simulink model "ControlNL"  (R2022b)
settings: Solver=ode45  StartTime=0.0  StopTime=1  RelTol=1e-3
values from neighbouring files (symbols this model uses):
  fceq = m*g    (= 20.601)    [Setup.m]
  J = diag([2.85e-6;2.85e-6;1.81e-6])    [Setup.m]
  m = 2.1    [Setup.m]
  MMA = [k1 k1 k1 k1 ... (first row only)    [Setup.m]
  Ts = 0.1    [Setup.m]
  x0 = [p0;v0;q0;omega0]    [Setup.m]
  xlin0 = [p0;v0;alpha0;omega0]    [Setup.m]
libraries: slpidlib x1
settings Model: Creator=stefanotonini  LastModifiedBy=stefanotonini

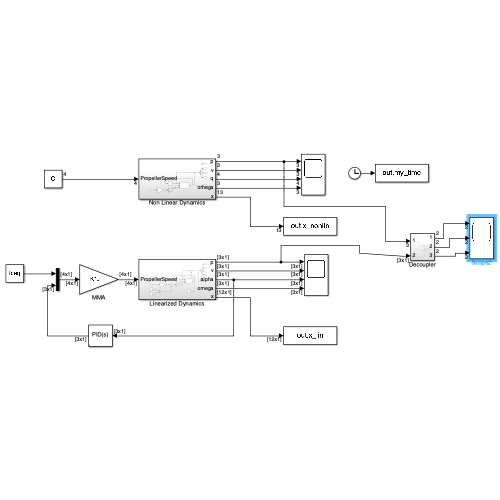
[thumbnail: Simulink's stored preview of the top-level diagram]
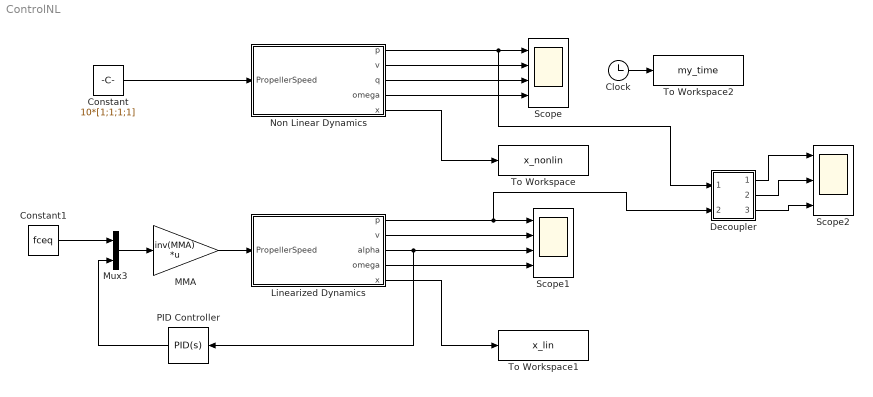
== system ControlNL ==
  Clock : Clock
  Constant : Constant  Value=10*[1;1;1;1]  SampleTime=Ts
  Constant1 : Constant  Value=fceq
  Decoupler : Subsystem
  Linearized Dynamics : Subsystem
  MMA : Gain  Gain=inv(MMA)  Multiplication=Matrix(K*u)
  Mux3 : Mux  Inputs=[1;3]
  Non Linear Dynamics : Subsystem
  PID Controller : slpidlib/PID Controller  Controller=PID  Form=Parallel  TimeDomain=Continuous-time  UseExternalTs=off  SampleTime=-1  IntegratorMethod=Forward Euler  FilterMethod=Forward Euler  ControllerParametersSource=internal  P=1  I=1  UseKiTs=off  D=0  N=100  UseFilter=on  TunerSelectOption=Transfer Function Based (PID Tuner App)  InitialConditionSource=internal  InitialConditionForIntegrator=0  InitialConditionForFilter=0  DifferentiatorICPrevScaledInput=0  ExternalReset=none  TrackingMode=off  Kt=1  LimitOutput=off  SatLimitsSource=internal  UpperSaturationLimit=inf  LowerSaturationLimit=-inf  LinearizeAsGain=on  AntiWindupMode=none  Kb=1  LimitIntegrator=off  UpperIntegratorSaturationLimit=inf  LowerIntegratorSaturationLimit=-inf  POutMin=[]  POutMax=[]  IOutMin=[]  IOutMax=[]  DOutMin=[]  DOutMax=[]  NOutMin=[]  NOutMax=[]  SumOutMin=[]  SumOutMax=[]  SaturationOutMin=[]  SaturationOutMax=[]  PParamMin=[]  PParamMax=[]  IParamMin=[]  IParamMax=[]  DParamMin=[]  DParamMax=[]  NParamMin=[]  NParamMax=[]  KbParamMin=[]  KbParamMax=[]  KtParamMin=[]  KtParamMax=[]  KbOutMin=[]  KbOutMax=[]  KtOutMin=[]  KtOutMax=[]  IntegratorOutMin=[]  IntegratorOutMax=[]  FilterOutMin=[]  FilterOutMax=[]  SumI1OutMin=[]  SumI1OutMax=[]  SumI2OutMin=[]  SumI2OutMax=[]  SumI3OutMin=[]  SumI3OutMax=[]  SumI4OutMin=[]  SumI4OutMax=[]  SumDOutMin=[]  SumDOutMax=[]  DifferentiatorOutMin=[]  DifferentiatorOutMax=[]  FilterDiffOutCoefMin=[]  FilterDiffOutCoefMax=[]  ReciprocalOutMin=[]  ReciprocalOutMax=[]  SumDenOutMin=[]  SumDenOutMax=[]  SumNumOutMin=[]  SumNumOutMax=[]  DivideOutMin=[]  DivideOutMax=[]  UdiffTsProdOutMin=[]  UdiffTsProdOutMax=[]  NTsProdOutMin=[]  NTsProdOutMax=[]  UintegralTsProdOutMin=[]  UintegralTsProdOutMax=[]  UngainTsProdOutMin=[]  UngainTsProdOutMax=[]  ClampingZeroOutDataTypeStr=Inherit: Inherit via back propagation  ClampingZeroOutMin=[]  ClampingZeroOutMax=[]  FilterDenConstantOutDataTypeStr=Inherit: Inherit via back propagation  FilterDenConstantOutMin=[]  FilterDenConstantOutMax=[]  PCopyOutDataTypeStr=Inherit: Inherit via back propagation  PCopyOutMin=[]  PCopyOutMax=[]  NCopyOutDataTypeStr=Inherit: Inherit via back propagation  NCopyOutMin=[]  NCopyOutMax=[]  IntegratorContinuousStateAttributes=''  IntegratorStateMustResolveToSignalObject=off  IntegratorRTWStateStorageClass=Auto  FilterContinuousStateAttributes=''  FilterStateMustResolveToSignalObject=off  FilterRTWStateStorageClass=Auto  ParallelPVariant=InternalParameters  IdealPVariant=Disabled  IVariant=InternalParameters  DVariant=InternalParameters  IntegratorVariant=Continuous  SatVariant=Disabled  AWVariant=Passthrough  PCopyVariant=Disabled  TRVariant=Disabled  FdbkBlocksVariant=Forward  IdealPFdbkVariant=Disabled  SatFdbkVariant=Disabled  DerivativeFilterVariant=ContFilter  NVariant=InternalParameters  NCopyVariant=Disabled  FilterICVariant=InternalICsFilter  IntegratorICVariant=InternalICs  ExternalResetVariant=Disabled  TRSumVariant=Passthrough  SumFdbkVariant=Disabled  SumVariant=Sum_PID  TsampFilterVariant=InternalTs  TsampNgainVariant=Passthrough  TsampIntegralVariant=Passthrough  ExternalSaturationOutDataTypeStr=Inherit: Same as second input
  Scope : Scope  NumInputPorts=4
  Scope1 : Scope  NumInputPorts=4
  Scope2 : Scope  NumInputPorts=3
  To Workspace : ToWorkspace  VariableName=x_nonlin  SampleTime=Ts
      settings: Save2DSignal=2-D array (concatenate along first dimension)
  To Workspace1 : ToWorkspace  VariableName=x_lin  SampleTime=Ts
      settings: Save2DSignal=2-D array (concatenate along first dimension)
  To Workspace2 : ToWorkspace  VariableName=my_time  SampleTime=Ts
      settings: Save2DSignal=2-D array (concatenate along first dimension)
  wires:
  Constant/1 -> Non Linear Dynamics/1(PropellerSpeed)
  Non Linear Dynamics/1(p) -> Decoupler/1(In1), Scope/1
  Non Linear Dynamics/2(v) -> Scope/2
  Non Linear Dynamics/3(q) -> Scope/3
  Non Linear Dynamics/4(omega) -> Scope/4
  Non Linear Dynamics/5(x) -> To Workspace/1
  Linearized Dynamics/5(x) -> To Workspace1/1
  Clock/1 -> To Workspace2/1
  Linearized Dynamics/1(p) -> Decoupler/2(In2), Scope1/1
  Linearized Dynamics/2(v) -> Scope1/2
  Linearized Dynamics/3(alpha) -> PID Controller/1, Scope1/3
  Linearized Dynamics/4(omega) -> Scope1/4
  Constant1/1 -> Mux3/1
  MMA/1 -> Linearized Dynamics/1(PropellerSpeed)
  Mux3/1 -> MMA/1
  PID Controller/1 -> Mux3/2
  Decoupler/1(Out1) -> Scope2/1
  Decoupler/2(Out2) -> Scope2/2
  Decoupler/3(Out3) -> Scope2/3

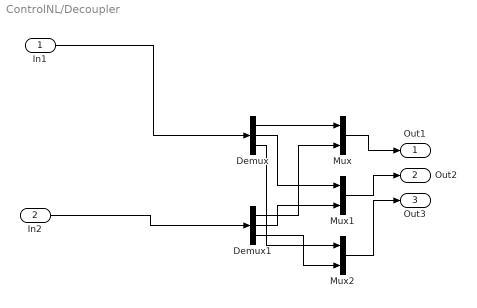
== system ControlNL/Decoupler ==
  In1 : Inport
  In2 : Inport  Port=2
  Demux : Demux  Outputs=3
  Demux1 : Demux  Outputs=3
  Mux : Mux  Inputs=2
  Mux1 : Mux  Inputs=2
  Mux2 : Mux  Inputs=2
  Out1 : Outport
  Out2 : Outport  Port=2
  Out3 : Outport  Port=3
  wires:
  In1/1 -> Demux/1
  Mux2/1 -> Out3/1
  Mux/1 -> Out1/1
  Demux/1 -> Mux/1
  Demux/2 -> Mux1/1
  Demux/3 -> Mux2/1
  Mux1/1 -> Out2/1
  Demux1/3 -> Mux2/2
  Demux1/1 -> Mux/2
  In2/1 -> Demux1/1
  Demux1/2 -> Mux1/2

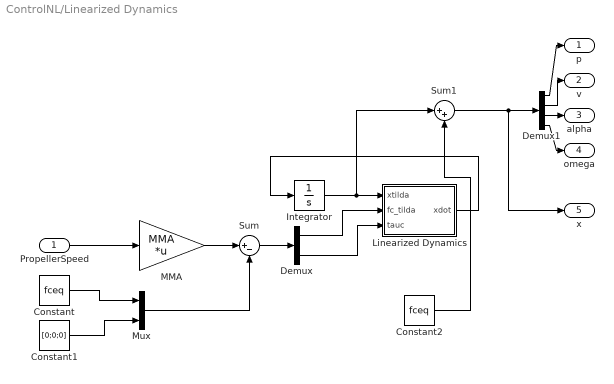
== system ControlNL/Linearized Dynamics ==
  PropellerSpeed : Inport
  Constant : Constant  Value=fceq
  Constant1 : Constant  Value=[0;0;0]
  Constant2 : Constant  Value=fceq
  Demux : Demux  Outputs=[1 3]
  Demux1 : Demux  Outputs=[3 3 3 3]
  Integrator : Integrator  InitialCondition=xlin0
  Linearized Dynamics : MATLAB Function  TreatAsAtomicUnit=on
  MMA : Gain  Gain=MMA  Multiplication=Matrix(K*u)
  Mux : Mux  Inputs=[1 3]
  Sum : Sum  Inputs=|+-
  Sum1 : Sum  Inputs=|++
  p : Outport
  v : Outport  Port=2
  alpha : Outport  Port=3
  omega : Outport  Port=4
  x : Outport  Port=5
  wires:
  PropellerSpeed/1 -> MMA/1
  Demux1/2 -> v/1
  Demux1/3 -> alpha/1
  Demux/1 -> Linearized Dynamics/2(fc_tilda)
  Demux1/4 -> omega/1
  Demux1/1 -> p/1
  Demux/2 -> Linearized Dynamics/3(tauc)
  Linearized Dynamics/1(xdot) -> Integrator/1
  Integrator/1 -> Sum1/1, Linearized Dynamics/1(xtilda)
  Constant/1 -> Mux/1
  Constant1/1 -> Mux/2
  Mux/1 -> Sum/2
  MMA/1 -> Sum/1
  Sum/1 -> Demux/1
  Sum1/1 -> x/1, Demux1/1
  Constant2/1 -> Sum1/2

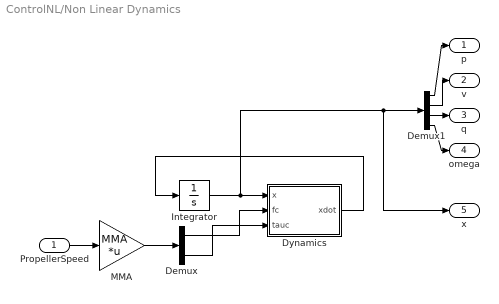
== system ControlNL/Non Linear Dynamics ==
  PropellerSpeed : Inport
  Demux : Demux  Outputs=[1 3]
  Demux1 : Demux  Outputs=[3 3 4 3]
  Dynamics : MATLAB Function  TreatAsAtomicUnit=on
  Integrator : Integrator  InitialCondition=x0
  MMA : Gain  Gain=MMA  Multiplication=Matrix(K*u)
  p : Outport
  v : Outport  Port=2
  q : Outport  Port=3
  omega : Outport  Port=4
  x : Outport  Port=5
  wires:
  PropellerSpeed/1 -> MMA/1
  Demux1/2 -> v/1
  Demux1/3 -> q/1
  Demux/1 -> Dynamics/2(fc)
  Demux1/4 -> omega/1
  Demux1/1 -> p/1
  Demux/2 -> Dynamics/3(tauc)
  Dynamics/1(xdot) -> Integrator/1
  Integrator/1 -> x/1, Demux1/1, Dynamics/1(x)
  MMA/1 -> Demux/1

== matlab function ControlNL/Non Linear Dynamics/Dynamics ==
  data: x input; fc input; xdot output size=13; tauc input; m parameter size=1; J parameter
function xdot = f(x,fc,tauc, m, J)

% Parameters
g = 9.81

% Extract State variables
p = x(1:3);
v = x(4:6);
q = x(7:10);
omega = x(11:13);
eta = q(1);
epsilon = q(2:4);


% Skew Matrix
S = [0 -q(4) -q(3);
    q(4) 0 -q(2);
    q(3) q(2) 0];
R = eye(3)+2*q(1)*S+2*S*S;

pdot = v;
vdot = m\([0;0;-m*g]+R*[0;0;fc]);

qdot = 1/2*[ -epsilon'*omega;
    (eta*eye(3)+S)*omega]
omegadot = J\(-cross(omega,J*omega)+tauc);

xdot = [pdot;vdot;qdot;omegadot];

== matlab function ControlNL/Linearized Dynamics/Linearized Dynamics ==
  data: xtilda input; fc_tilda input; xdot output; tauc input; m parameter size=1; J parameter; fceq parameter
function xdot = f(xtilda,fc_tilda,tauc, m, J, fceq)

% Extract State variables
p_tilda = xtilda(1:3);
v_tilda = xtilda(4:6);
alpha_tilda = xtilda(7:9);
omega_tilda = xtilda(10:12);

phi_tilda = alpha_tilda(1); % Roll
theta_tilda = alpha_tilda(2); % Pitch
psi_tilda = alpha_tilda(3); % Yaw


pdot = v_tilda;
vdot = m\([fceq*theta_tilda; -fceq*phi_tilda; fc_tilda]);

alphadot = omega_tilda;

omegadot = J\(tauc);

xdot = [pdot;vdot;alphadot;omegadot];
